simulink model "rct_helico_Zdomain"  (R2018a)
settings: Solver=ode23t  StartTime=0.0  StopTime=10.0  MaxStep=0.001  RelTol=1e-6
model workspace (MAT data in the model file):
  A = [-0.0191  0.017  0.3839  -9.7924  -0.0008  -0.3371  0  0; 0.0136  -0.2994  0.0237  -0.5859  -0.0017  -0.0257  0.5374  0; 0.0405  -0.0026  -1.8394  0  0.0024  0.5281  0  -0.0015; 0  0  0.9985  0  0  0  0  0.0549; 0.001  -0.0017  -0.3381  0.0322  -0.0349  -0.4032  9.7777  0.1168; 0.013  0  -3.047  0  -0.229  -10.6199  0  -0.0333; 0  0  -0.0033  0  0  1  0  0.0598; 0.002  0.006  -0.5412  0  0.0039  -1.8554  0  -0.3487]
  B = [-10.3456  1.0793  0; -0.7293  0.0755  0; 27.09  -4.7239  -0.1857; 0  0  0; -1.082  -10.3713  4.7239; -27.2884  -156.4425  -1.069; 0  0  0; -4.8969  -27.9728  -12.9304]
  Cmeas = [0  0  0  1  0  0  0  0; 0  0  0  0  0  0  1  0; 0  0  0  0  0  0  0  1; 0  0  1  0  0  0  0  0; 0  0  0  0  0  1  0  0]
libraries: simulink x1
settings Model: FPTRunName=Active  Creator=The MathWorks Inc.  LastModifiedBy=bpotter
settings DataIOCC: LimitDataPoints=on  SaveFormat=Array
settings OptimizationCC: BlockReduction=off  BooleanDataType=off  LifeSpan=inf
settings DebuggingCC: SaveWithParameterizedLinksMsg=none  UnderspecifiedInitializationDetection=Classic  MergeDetectMultiDrivingBlocksExec=none  SignalResolutionControl=TryResolveAllWithWarning  AllowSymbolicDim=off  StrictBusMsg=ErrorOnBusTreatedAsVector  NonBusSignalsTreatedAsBus=error  SFUnexpectedBacktrackingDiag=warning  SFNoUnconditionalDefaultTransitionDiag=warning  SFExecutionAtInitializationDiag=none
settings HardwareCC: ProdBitPerPointer=32  ProdBitPerSizeT=32  ProdBitPerPtrDiffT=32  ProdLargestAtomicFloat=None  ProdEndianess=Unspecified  ProdWordSize=32  ProdHWDeviceType=32-bit Generic  TargetUnknown=on
settings ModelReferenceCC: PropagateSignalLabelsOutOfModel=off
settings CodeAppCC: StateflowObjectComments=on
settings GRTTargetCC: TargetLangStandard=C89/C90 (ANSI)  GeneratePreprocessorConditionals=Disable all
settings ConfigComp: CovMetricSettings=dw  CovHtmlReporting=on  CovSaveCumulativeToWorkspaceVar=on  CovSaveSingleToWorkspaceVar=on  CovExternalEMLEnable=off

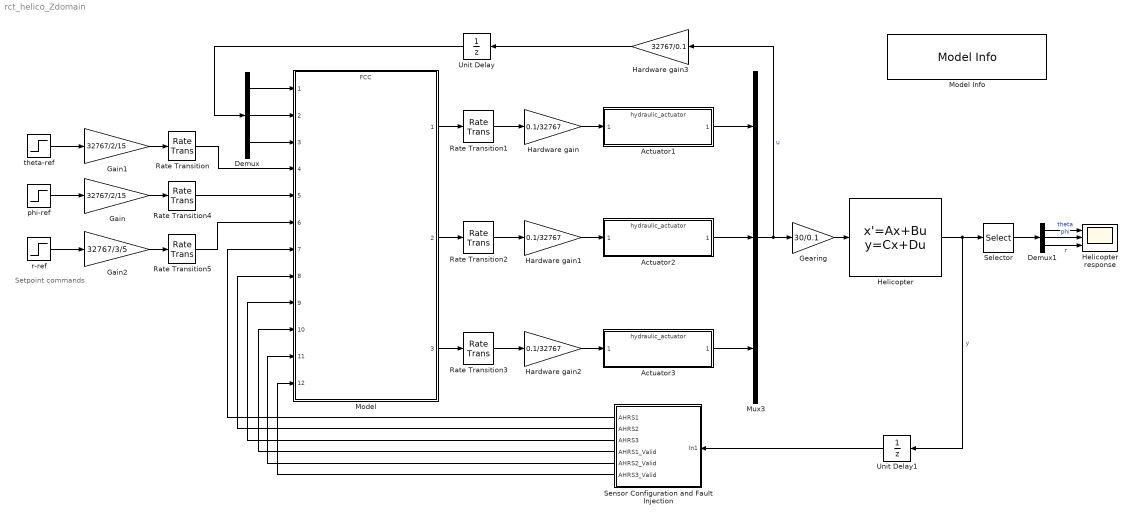
== system rct_helico_Zdomain ==
  note: Setpoint
      | commands
  Actuator1 : ModelReference  ModelNameDialog=hydraulic_actuator  ModelReferenceVersion=1.87
  Actuator2 : ModelReference  ModelNameDialog=hydraulic_actuator  ModelReferenceVersion=1.87
  Actuator3 : ModelReference  ModelNameDialog=hydraulic_actuator  ModelReferenceVersion=1.87
  Demux : Demux  Outputs=3
  Demux1 : Demux  Outputs=3
  Gain : Gain  Gain=32767/2/15  OutDataTypeStr=int16
  Gain1 : Gain  Gain=32767/2/15  OutDataTypeStr=int16
  Gain2 : Gain  Gain=32767/3/5  OutDataTypeStr=int16
  Gearing : Gain  Gain=30/0.1
  Hardware gain : Gain  Gain=0.1/32767  OutDataTypeStr=double
  Hardware gain1 : Gain  Gain=0.1/32767  OutDataTypeStr=double
  Hardware gain2 : Gain  Gain=0.1/32767  OutDataTypeStr=double
  Hardware gain3 : Gain  Gain=32767/0.1  OutDataTypeStr=int16  SaturateOnIntegerOverflow=on
  Helicopter : StateSpace  A=A  B=B  C=Cmeas  D=zeros(5,3)  InitialCondition=0
      mask Display: image('helicopter.jpg');
  Helicopter response : Scope  NumInputPorts=3
  Model : ModelReference  ModelNameDialog=FCC  SimulationMode=Normal  ModelReferenceVersion=1.50
  Model Info : simulink/Model-Wide Utilities/Model Info  Frame=on  DisplayStringWithTags=|  HorizontalTextAlignment=Center  LeftAlignmentValue=0.5
      | Model: %<ModelName>
      | Model Version: %<ModelVersion>
      | Last Modified: %<LastModificationDate>
      | 
      | Copyright 2016 The MathWorks, Inc.
  Mux3 : Mux  Inputs=3
  Rate Transition : RateTransition  OutPortSampleTime=0.01
  Rate Transition1 : RateTransition  OutPortSampleTime=0.001
  Rate Transition2 : RateTransition  OutPortSampleTime=0.001
  Rate Transition3 : RateTransition  OutPortSampleTime=0.001
  Rate Transition4 : RateTransition  OutPortSampleTime=0.01
  Rate Transition5 : RateTransition  OutPortSampleTime=0.01
  Selector : Selector  InputPortWidth=5  IndexOptions=Index vector (dialog)  Indices=[1 2 3]  OutputSizes=1
  Sensor Configuration and Fault Injection : Subsystem  TreatAsAtomicUnit=on
  Unit Delay : UnitDelay  SampleTime=0.001
  Unit Delay1 : UnitDelay  SampleTime=0.001
  phi-ref : Step  Time=3  SampleTime=0
  r-ref : Step  Time=6  SampleTime=0
  theta-ref : Step  Time=0  SampleTime=0
  wires:
  Helicopter/1 -> Unit Delay1/1, Selector/1  "y"
  Mux3/1 -> Hardware gain3/1, Gearing/1  "u"
  Selector/1 -> Demux1/1
  Demux1/1 -> Helicopter response/1  "theta"
  Demux1/2 -> Helicopter response/2  "phi"
  Demux1/3 -> Helicopter response/3  "r"
  Actuator1/1 -> Mux3/1
  Actuator3/1 -> Mux3/3
  Actuator2/1 -> Mux3/2
  theta-ref/1 -> Gain1/1
  phi-ref/1 -> Gain/1
  r-ref/1 -> Gain2/1
  Model/1 -> Rate Transition1/1
  Rate Transition1/1 -> Hardware gain/1
  Rate Transition3/1 -> Hardware gain2/1
  Model/3 -> Rate Transition3/1
  Model/2 -> Rate Transition2/1
  Rate Transition2/1 -> Hardware gain1/1
  Demux/2 -> Model/2
  Demux/1 -> Model/1
  Demux/3 -> Model/3
  Unit Delay/1 -> Demux/1
  Gearing/1 -> Helicopter/1
  Unit Delay1/1 -> Sensor Configuration and Fault Injection/1(In1)
  Sensor Configuration and Fault Injection/1(AHRS1) -> Model/7
  Sensor Configuration and Fault Injection/2(AHRS2) -> Model/8
  Sensor Configuration and Fault Injection/3(AHRS3) -> Model/9
  Sensor Configuration and Fault Injection/4(AHRS1_Valid) -> Model/10
  Sensor Configuration and Fault Injection/5(AHRS2_Valid) -> Model/11
  Sensor Configuration and Fault Injection/6(AHRS3_Valid) -> Model/12
  Hardware gain/1 -> Actuator1/1
  Hardware gain1/1 -> Actuator2/1
  Hardware gain2/1 -> Actuator3/1
  Hardware gain3/1 -> Unit Delay/1
  Rate Transition/1 -> Model/4
  Gain1/1 -> Rate Transition/1
  Gain/1 -> Rate Transition4/1
  Rate Transition4/1 -> Model/5
  Gain2/1 -> Rate Transition5/1
  Rate Transition5/1 -> Model/6

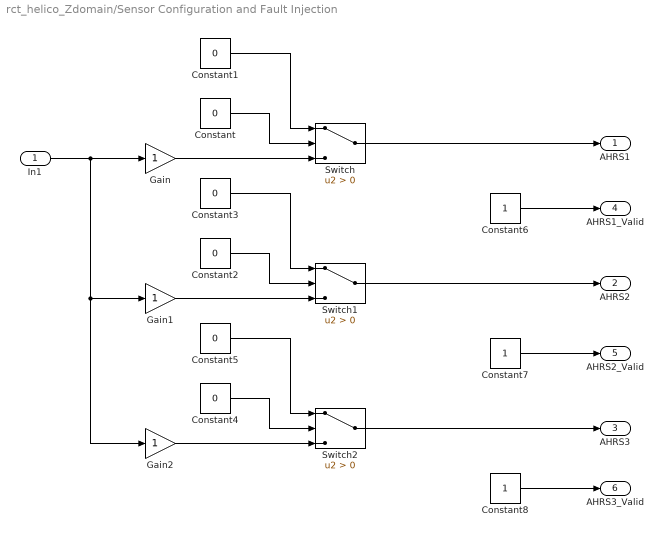
== system rct_helico_Zdomain/Sensor Configuration and Fault Injection ==
  In1 : Inport
  Constant{,1..5} (6 alike) : Constant  Value=0
  Constant6 : Constant  OutDataTypeStr=boolean
  Constant7 : Constant  OutDataTypeStr=boolean
  Constant8 : Constant  OutDataTypeStr=boolean
  Gain : Gain
  Gain1 : Gain
  Gain2 : Gain
  Switch : Switch  Criteria=u2 > Threshold
  Switch1 : Switch  Criteria=u2 > Threshold
  Switch2 : Switch  Criteria=u2 > Threshold
  AHRS1 : Outport
  AHRS2 : Outport  Port=2
  AHRS3 : Outport  Port=3
  AHRS1_Valid : Outport  Port=4
  AHRS2_Valid : Outport  Port=5
  AHRS3_Valid : Outport  Port=6
  wires:
  In1/1 -> Gain1/1, Gain2/1, Gain/1
  Gain/1 -> Switch/3
  Constant/1 -> Switch/2
  Constant1/1 -> Switch/1
  Switch/1 -> AHRS1/1
  Gain1/1 -> Switch1/3
  Constant2/1 -> Switch1/2
  Constant3/1 -> Switch1/1
  Gain2/1 -> Switch2/3
  Constant4/1 -> Switch2/2
  Constant5/1 -> Switch2/1
  Switch1/1 -> AHRS2/1
  Switch2/1 -> AHRS3/1
  Constant6/1 -> AHRS1_Valid/1
  Constant7/1 -> AHRS2_Valid/1
  Constant8/1 -> AHRS3_Valid/1
